simulink model "DataValueAndQualityIndicator"  (R2025a)
settings: Solver=VariableStepAuto  StartTime=0.0  StopTime=inf  MaxStep=0.01  RelTol=1e-3
undefined symbols (not defined in the file): DiscIntNeverNeededParam
libraries: opcualib x2
settings Model: Creator=The MathWorks, Inc.  LastModifiedBy=noast

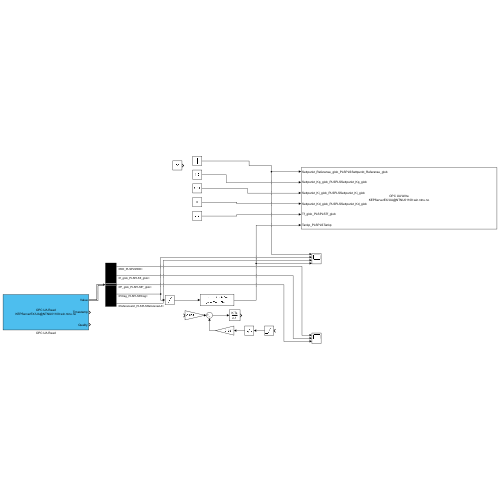
[thumbnail: Simulink's stored preview of the top-level diagram]
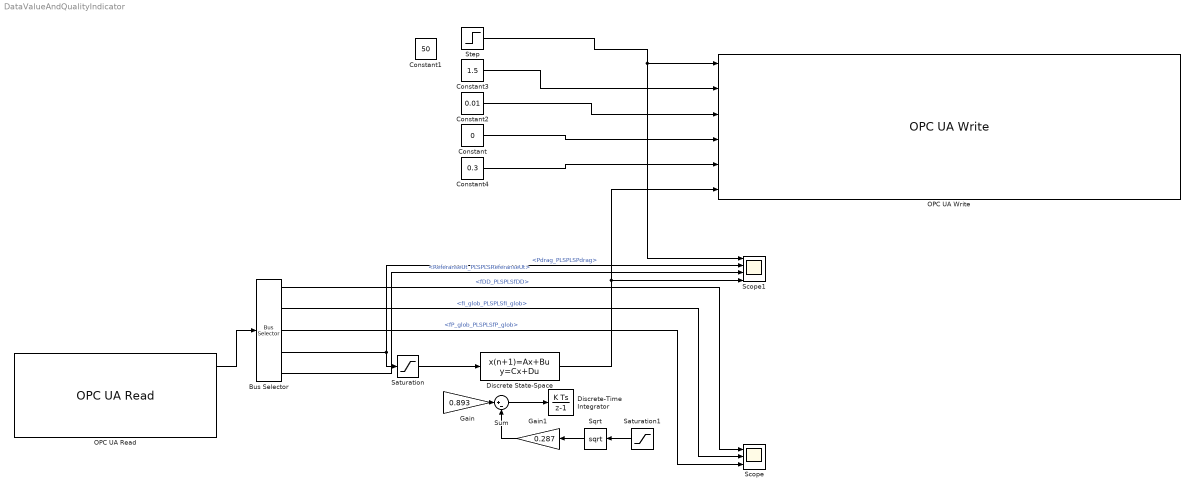
== system DataValueAndQualityIndicator ==
  Bus Selector : BusSelector  OutputSignals=fDD_PLSPLSfDD,fI_glob_PLSPLSfI_glob,fP_glob_PLSPLSfP_glob,Pdrag_PLSPLSPdrag,ReferanseUt_PLSPLSReferanseUt
  Constant : Constant  Value=0
  Constant1 : Constant  Value=50
  Constant2 : Constant  Value=0.01
  Constant3 : Constant  Value=1.5
  Constant4 : Constant  Value=0.3
  Discrete State-Space : DiscreteStateSpace  A=0.999841  B=0.001587  D=0  InitialCondition=40  SampleTime=-1
  Discrete-Time Integrator : DiscreteIntegrator  SampleTime=-1  ICPrevOutput=DiscIntNeverNeededParam  ICPrevScaledInput=DiscIntNeverNeededParam
  Gain : Gain  Gain=0.893
  Gain1 : Gain  Gain=0.287
  OPC UA Read : opcualib/OPC UA Read  Priority=2  SelectedServer=KEPServerEX/UA@NTNU01109.win.ntnu.no  ServerList=KEPServerEX/UA@NTNU01109.win.ntnu.no  NodeList={ '1', 'fDD', '2', 'PLS.PLS.fDD', '0'; '2', 'fI_glob', '2', 'PLS.PLS.fI_glob', '0'; '3', 'fP_glob', '2', 'PLS.PLS.fP_glob', '0'; '4', 'Pådrag', '2', 'PLS.PLS.Pådrag', '0'; '5', 'Referanse Ut', '2', 'PLS.PLS.Referanse Ut', '0' }  ShowQualityPort=on  ShowTimestampPort=on  ShowTimestampPortAs=Seconds since start  SampleTime=-1
      settings: LibrarySourceBlock=abc/MATLAB System
  OPC UA Write : opcualib/OPC UA Write  SelectedServer=KEPServerEX/UA@NTNU01109.win.ntnu.no  ServerList=KEPServerEX/UA@NTNU01109.win.ntnu.no  SampleTime=-1  NodeList={ '1', 'Settpunkt_Referanse_glob', '2', 'PLS.PLS.Settpunkt_Referanse_glob', '0'; '2', 'Settpunkt_Kp_glob', '2', 'PLS.PLS.Settpunkt_Kp_glob', '0'; '3', 'Settpunkt_Ki_glob', '2', 'PLS.PLS.Settpunkt_Ki_glob', '0'; '4', 'Settpunkt_Kd_glob', '2', 'PLS.PLS.Settpunkt_Kd_glob', '0'; '5', 'Tf_glob', '2', 'PLS.PLS.Tf_glob', '0'; '6', 'Tankp', '2', 'PLS.PLS.Tankp', '0' }
  Saturation : Saturate  UpperLimit=100  LowerLimit=0
  Saturation1 : Saturate  UpperLimit=50  LowerLimit=0
  Scope : Scope  NumInputPorts=3
      settings: ActiveDisplayYMinimum=-19.675948619842526  ActiveDisplayYMaximum=135.51954984664917
  Scope1 : Scope  NumInputPorts=4
      settings: ActiveDisplayYMinimum=-7.5938808321952784  ActiveDisplayYMaximum=111.9548756480217
  Sqrt : Sqrt
  Step : Step  Before=40  After=50  SampleTime=0
  Sum : Sum  Inputs=|+-
  wires:
  Discrete State-Space/1 -> OPC UA Write/6, Scope1/4
  Constant4/1 -> OPC UA Write/5
  Constant3/1 -> OPC UA Write/2
  Constant2/1 -> OPC UA Write/3
  Step/1 -> OPC UA Write/1, Scope1/1
  Constant/1 -> OPC UA Write/4
  Saturation/1 -> Discrete State-Space/1
  Sum/1 -> Discrete-Time Integrator/1
  Bus Selector/4 -> Saturation/1, Scope1/2  "<Pdrag_PLSPLSPdrag>"
  Bus Selector/1 -> Scope/1  "<fDD_PLSPLSfDD>"
  Bus Selector/2 -> Scope/2  "<fI_glob_PLSPLSfI_glob>"
  Bus Selector/3 -> Scope/3  "<fP_glob_PLSPLSfP_glob>"
  Gain/1 -> Sum/1
  Sqrt/1 -> Gain1/1
  Gain1/1 -> Sum/2
  Saturation1/1 -> Sqrt/1
  OPC UA Read/1 -> Bus Selector/1
  Bus Selector/5 -> Scope1/3  "<ReferanseUt_PLSPLSReferanseUt>"
